simulink model "DoubleLeafWall"  (R2021b)
settings: Solver=ode45  StartTime=0.0  StopTime=60  RelTol=1e-3
values from neighbouring files (symbols this model uses):
  c = 3    [plotX2vsW.m]    (also in plotX2vsWLowerFreq.m; plotX2vsWaddedCw.m; simulateX2vsWaddedCa.m)
  ca = caList(simNum)    [simulateX2vsWaddedCa.m]
  cw = 500    [plotX2vsWaddedCw.m]    (also in simulateX2vsWaddedCa.m)
  F = 10    [plotX2vsW.m]    (also in plotX2vsWLowerFreq.m; plotX2vsWaddedCw.m; simulateX2vsWaddedCa.m)
  k = 171080    [plotX2vsW.m]    (also in plotX2vsWLowerFreq.m; plotX2vsWaddedCw.m; simulateX2vsWaddedCa.m)
  ka = 34222.5    [simulateX2vsWaddedCa.m]
  m1 = 1    [plotX2vsW.m]    (also in plotX2vsWLowerFreq.m; plotX2vsWaddedCw.m; simulateX2vsWaddedCa.m)
  m2 = 1    [plotX2vsW.m]    (also in plotX2vsWLowerFreq.m; plotX2vsWaddedCw.m; simulateX2vsWaddedCa.m)
  ma = 0.1    [simulateX2vsWaddedCa.m]
  w = zeros(815,1)    [plotX2vsW.m]    (also in plotX2vsWLowerFreq.m = zeros(175,1); plotX2vsWaddedCw.m; simulateX2vsWaddedCa.m = 125:5:940)
settings Model: Creator=vsor436  LastModifiedBy=bl4ck
settings SolverCC: AlgebraicLoopSolver=TrustRegion
settings DebuggingCC: SFMachineParentedDataDiag=warning

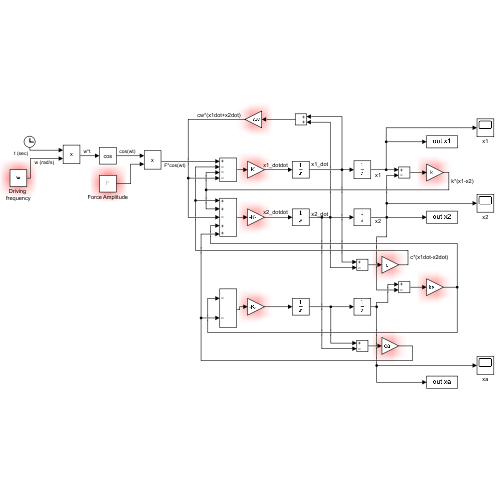
[thumbnail: Simulink's stored preview of the top-level diagram]
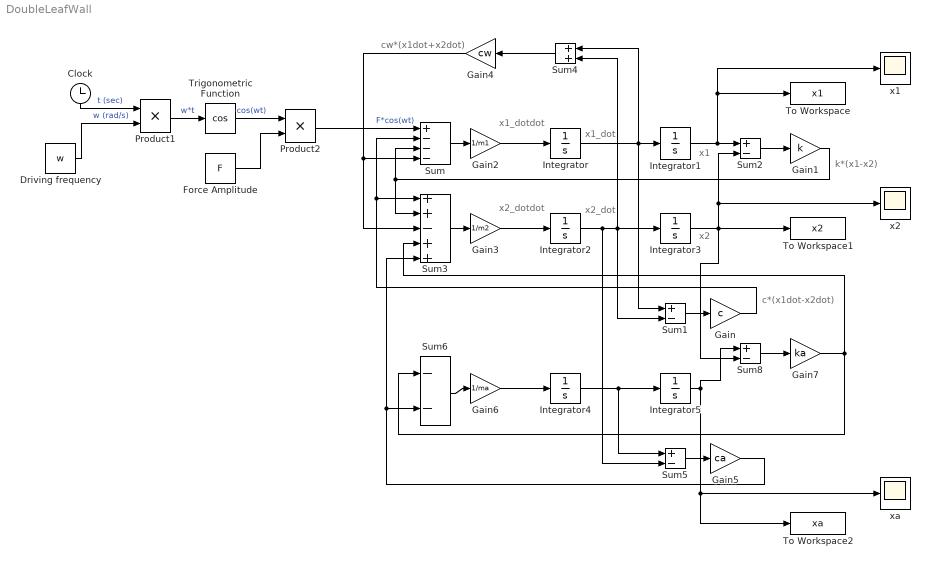
== system DoubleLeafWall ==
  note: k*(x1-x2)
  note: cw*(x1dot+x2dot)
  note: c*(x1dot-x2dot)
  note: x1_dotdot
  note: x2
  note: x1
  note: x1_dot
  note: x2_dot
  note: x2_dotdot
  Clock : Clock
  Driving frequency : Constant  Value=w
  Force Amplitude : Constant  Value=F
  Gain : Gain  Gain=c
  Gain1 : Gain  Gain=k
  Gain2 : Gain  Gain=1/m1
  Gain3 : Gain  Gain=1/m2
  Gain4 : Gain  Gain=cw
  Gain5 : Gain  Gain=ca
  Gain6 : Gain  Gain=1/ma
  Gain7 : Gain  Gain=ka
  Integrator{,2..5} (5 alike) : Integrator
  Integrator1 : Integrator  UpperSaturationLimit=0.01  LowerSaturationLimit=-0.01  WrappedStateUpperValue=0.01  WrappedStateLowerValue=-0.01
  Product1 : Product
  Product2 : Product
  Sum : Sum  Inputs=+---
  Sum{1..2,5,8} (4 alike) : Sum  Inputs=+-
  Sum3 : Sum  Inputs=++-++
  Sum4 : Sum
  Sum6 : Sum  Inputs=--
  To Workspace : ToWorkspace  VariableName=x1  SampleTime=-1
  To Workspace1 : ToWorkspace  VariableName=x2  SampleTime=-1
  To Workspace2 : ToWorkspace  VariableName=xa  SampleTime=-1
  Trigonometric Function : Trigonometry  Operator=cos
  x1 : Scope
  x2 : Scope
  xa : Scope
  wires:
  Product1/1 -> Trigonometric Function/1  "w*t"
  Trigonometric Function/1 -> Product2/1  "cos(wt)"
  Clock/1 -> Product1/1  "t (sec)"
  Driving frequency/1 -> Product1/2  "w (rad/s)"
  Force Amplitude/1 -> Product2/2
  Product2/1 -> Sum/1  "F*cos(wt)"
  Integrator/1 -> Sum1/1, Sum4/1, Integrator1/1
  Sum1/1 -> Gain/1
  Gain/1 -> Sum/2, Sum3/1
  Sum2/1 -> Gain1/1
  Gain1/1 -> Sum/3, Sum3/2
  Sum/1 -> Gain2/1
  Gain2/1 -> Integrator/1
  Gain3/1 -> Integrator2/1
  Sum3/1 -> Gain3/1
  Integrator1/1 -> x1/1, To Workspace/1, Sum2/1
  Integrator3/1 -> Sum8/2, To Workspace1/1, Sum2/2, x2/1
  Integrator2/1 -> Sum5/2, Sum4/2, Integrator3/1, Sum1/2
  Sum4/1 -> Gain4/1
  Gain4/1 -> Sum3/3, Sum/4
  Sum5/1 -> Gain5/1
  Sum6/1 -> Gain6/1
  Gain6/1 -> Integrator4/1
  Integrator4/1 -> Sum5/1, Integrator5/1
  Integrator5/1 -> Sum8/1, xa/1, To Workspace2/1
  Sum8/1 -> Gain7/1
  Gain7/1 -> Sum3/4, Sum6/1
  Gain5/1 -> Sum3/5, Sum6/2
